simulink model "untitled"  (R2021a)
settings: Solver=FixedStepAuto  StartTime=0.0  StopTime=inf  RelTol=1e-3  EnableMultiTasking=on
libraries: pil_lib x1
settings Model: Creator=Abbas  LastModifiedBy=Abbas
settings OptimizationCC: EnhancedBackFolding=on  PassReuseOutputArgsAs=Individual arguments  ZeroExternalMemoryAtStartup=off  ZeroInternalMemoryAtStartup=off  MaxStackSize=64  OptimizeBlockOrder=speed  DifferentSizesBufferReuse=on  OptimizationCustomize=off  EfficientTunableParamExpr=on
settings DebuggingCC: ParameterTunabilityLossMsg=error
settings HardwareCC: ProdBitPerInt=16  ProdBitPerPointer=16  ProdBitPerSizeT=16  ProdBitPerPtrDiffT=16  ProdLargestAtomicFloat=None  ProdWordSize=8  ProdHWDeviceType=Atmel->AVR
settings SFSimCC: MATLABDynamicMemAlloc=off
settings RTWCC: SystemTargetFile=ert.tlc  HardwareBoard=Arduino Mega 2560  TemplateMakefile=ert_default_tmf  Toolchain=Arduino AVR  BuildConfiguration=Faster Runs  CreateSILPILBlock=PIL
settings CodeAppCC: ForceParamTrailComments=on  IgnoreCustomStorageClasses=off  OperatorAnnotations=on  SimulinkDataObjDesc=on  SFDataObjDesc=on  InsertBlockDesc=on
settings ERTTargetCC: SupportContinuousTime=on  SupportVariableSizeSignals=on  ExtModeStaticAllocSize=2048

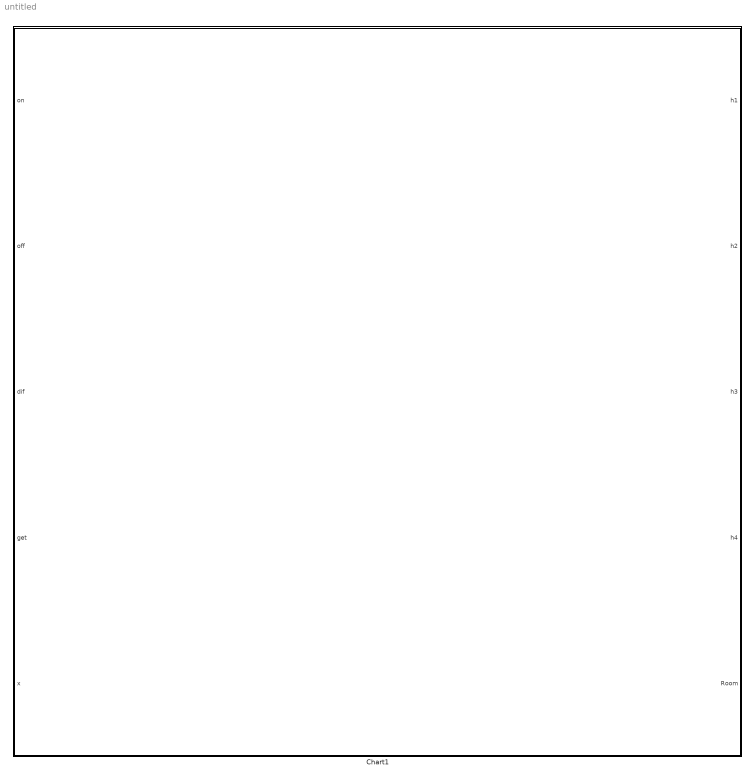
== system untitled ==
  Chart1 : Subsystem  DialogController=pil_create_dialog  LoadFcn=|
      | try
      |    if ~strcmp(rtw.pil.getPILVersion, '9.10 (R2021a)_15')
      |       set_param(gcb, 'DialogController', '');
      |       set_param(gcb, 'DialogControllerArgs', '');
      |    end
      | catch e
      |       set_param(gcb, 'DialogController', '');
      |       set_param(gcb, 'DialogControllerArgs', '');
      | end
      mask help: PIL:pil:XILBlockMaskDesc
      mask Display: disp('PIL');

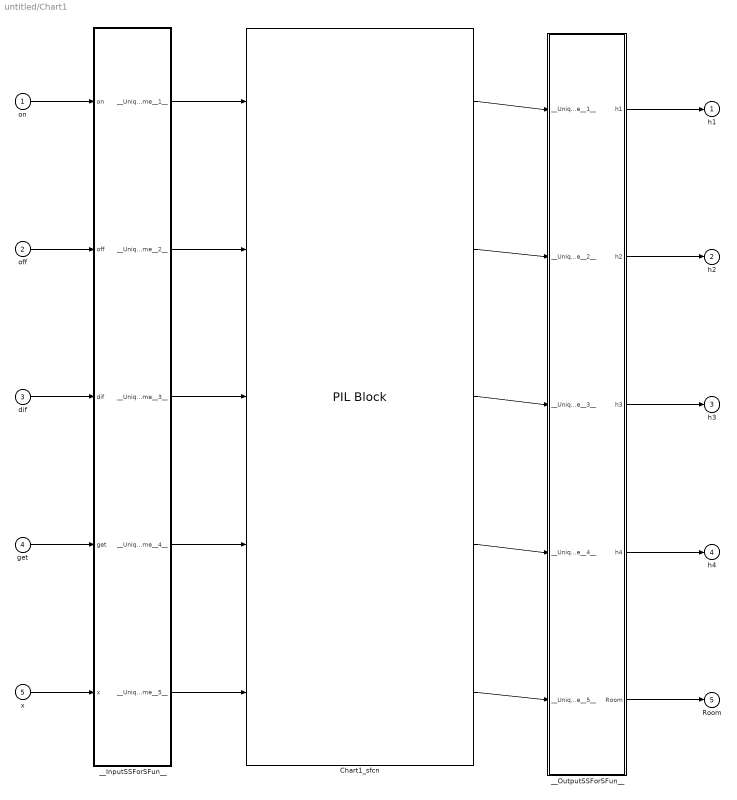
== system untitled/Chart1 ==
  on : Inport
  off : Inport  Port=2
  dif : Inport  Port=3
  get : Inport  Port=4
  x : Inport  Port=5
  Chart1_sfcn : pil_lib/PIL Block  SimulationMode=PIL  IsTopModelPIL=off  CodeDir=C:\test2\Chart1_ert_rtw  AnchorDir=C:\test2  ConfigName=Arduino Board  XrelIsTopModelCode=on  XrelIsReusable=off  XrelDWorkNames={}  XrelDWorkTypes={}  XrelModelArgVals={}  XrelOrderedParamNames={}
      settings: SourceProductBaseCode=RT
  __InputSSForSFun__ : Subsystem
  __OutputSSForSFun__ : Subsystem
  h1 : Outport
  h2 : Outport  Port=2
  h3 : Outport  Port=3
  h4 : Outport  Port=4
  Room : Outport  Port=5
  wires:
  on/1 -> __InputSSForSFun__/1(on)
  off/1 -> __InputSSForSFun__/2(off)
  dif/1 -> __InputSSForSFun__/3(dif)
  get/1 -> __InputSSForSFun__/4(get)
  x/1 -> __InputSSForSFun__/5(x)
  __InputSSForSFun__/1(__UniqueOutportName__1__) -> Chart1_sfcn/1
  __InputSSForSFun__/2(__UniqueOutportName__2__) -> Chart1_sfcn/2
  __InputSSForSFun__/3(__UniqueOutportName__3__) -> Chart1_sfcn/3
  __InputSSForSFun__/4(__UniqueOutportName__4__) -> Chart1_sfcn/4
  __InputSSForSFun__/5(__UniqueOutportName__5__) -> Chart1_sfcn/5
  Chart1_sfcn/1 -> __OutputSSForSFun__/1(__UniqueInportName__1__)
  Chart1_sfcn/2 -> __OutputSSForSFun__/2(__UniqueInportName__2__)
  Chart1_sfcn/3 -> __OutputSSForSFun__/3(__UniqueInportName__3__)
  Chart1_sfcn/4 -> __OutputSSForSFun__/4(__UniqueInportName__4__)
  Chart1_sfcn/5 -> __OutputSSForSFun__/5(__UniqueInportName__5__)
  __OutputSSForSFun__/1(h1) -> h1/1
  __OutputSSForSFun__/2(h2) -> h2/1
  __OutputSSForSFun__/3(h3) -> h3/1
  __OutputSSForSFun__/4(h4) -> h4/1
  __OutputSSForSFun__/5(Room) -> Room/1

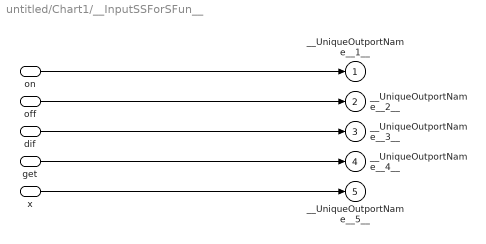
== system untitled/Chart1/__InputSSForSFun__ ==
  on : Inport
  off : Inport  Port=2
  dif : Inport  Port=3
  get : Inport  Port=4
  x : Inport  Port=5
  __UniqueOutportName__1__ : Outport
  __UniqueOutportName__2__ : Outport  Port=2
  __UniqueOutportName__3__ : Outport  Port=3
  __UniqueOutportName__4__ : Outport  Port=4
  __UniqueOutportName__5__ : Outport  Port=5
  wires:
  on/1 -> __UniqueOutportName__1__/1
  off/1 -> __UniqueOutportName__2__/1
  dif/1 -> __UniqueOutportName__3__/1
  get/1 -> __UniqueOutportName__4__/1
  x/1 -> __UniqueOutportName__5__/1

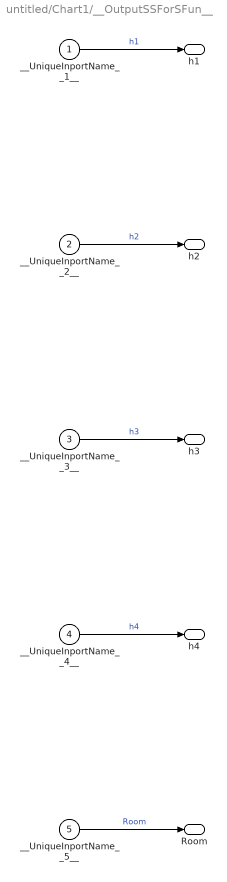
== system untitled/Chart1/__OutputSSForSFun__ ==
  __UniqueInportName__1__ : Inport
  __UniqueInportName__2__ : Inport  Port=2
  __UniqueInportName__3__ : Inport  Port=3
  __UniqueInportName__4__ : Inport  Port=4
  __UniqueInportName__5__ : Inport  Port=5
  h1 : Outport
  h2 : Outport  Port=2
  h3 : Outport  Port=3
  h4 : Outport  Port=4
  Room : Outport  Port=5
  wires:
  __UniqueInportName__1__/1 -> h1/1  "h1"
  __UniqueInportName__2__/1 -> h2/1  "h2"
  __UniqueInportName__3__/1 -> h3/1  "h3"
  __UniqueInportName__4__/1 -> h4/1  "h4"
  __UniqueInportName__5__/1 -> Room/1  "Room"
